simulink subsystem "FTC2019b"  (R2019b)
settings: Solver=VariableStepAuto  StartTime=0.0  StopTime=10.0  RelTol=1e-3
values from neighbouring files (symbols this model uses):
  g = (9.8)    (= 9.8)    [H250_LOEKnown_400HzParam.m]    (also in H250_LOEUnknown_400HzParam.m; H333_LOEKnown_400HzParam.m)
  J = (diag([0.0056 0.0056 0.0104]))    [H250_LOEKnown_400HzParam.m]    (also in H250_LOEUnknown_400HzParam.m; H333_LOEKnown_400HzParam.m = (diag([0.012 0.0120 0.02])))
  m = (0.752)    (= 0.752)    [H250_LOEKnown_400HzParam.m]    (also in H250_LOEUnknown_400HzParam.m; H333_LOEKnown_400HzParam.m = 1.13)
  M = ([ 1          1          1         1 ... (first row only)    [H250_LOEKnown_400HzParam.m]    (also in H250_LOEUnknown_400HzParam.m; H333_LOEKnown_400HzParam.m)
  MY_ATT_P = Pixhawk_CSC.Parameter( {single(8), 'MY_ATT_P'}  )    [H250_LOEKnown_400HzParam.m]    (also in H250_LOEUnknown_400HzParam.m = Pixhawk_CSC.Parameter( {single(3), 'MY_ATT_P'}  ); H333_LOEKnown_400HzParam.m)
  MY_ATT_P_YAW = Pixhawk_CSC.Parameter( {single(0), 'MY_ATT_P_YAW'}  )    [H250_LOEKnown_400HzParam.m]    (also in H250_LOEUnknown_400HzParam.m = Pixhawk_CSC.Parameter( {single(0.0), 'MY_ATT_P_YAW'}  ); H333_LOEKnown_400HzParam.m)
  MY_POS_P = Pixhawk_CSC.Parameter( {single(0.5), 'MY_POS_P'}  )    [H250_LOEKnown_400HzParam.m]    (also in H250_LOEUnknown_400HzParam.m; H333_LOEKnown_400HzParam.m)
  MY_RATE_P = Pixhawk_CSC.Parameter( {single(12), 'MY_RATE_P'}  )    [H250_LOEKnown_400HzParam.m]    (also in H250_LOEUnknown_400HzParam.m = Pixhawk_CSC.Parameter( {single(14), 'MY_RATE_P'}  ); H333_LOEKnown_400HzParam.m)
  MY_RATE_P_YAW = Pixhawk_CSC.Parameter( {single(0.3), 'MY_RATE_P_YAW'}  )    [H250_LOEKnown_400HzParam.m]    (also in H250_LOEUnknown_400HzParam.m = Pixhawk_CSC.Parameter( {single(0.0), 'MY_RATE_P_YAW'}  ); H333_LOEKnown_400HzParam.m)
  MY_SAT_AD = Pixhawk_CSC.Parameter({single(0.13), 'MY_SAT_AD'} )    [H250_LOEKnown_400HzParam.m]    (also in H250_LOEUnknown_400HzParam.m; H333_LOEKnown_400HzParam.m)
  MY_TAU_P_A = Pixhawk_CSC.Parameter( {single(0), 'MY_TAU_P_A'}  )    [H250_LOEKnown_400HzParam.m]    (also in H250_LOEUnknown_400HzParam.m = Pixhawk_CSC.Parameter( {single(0.0), 'MY_TAU_P_A'}  ); H333_LOEKnown_400HzParam.m)
  MY_TAU_P_A_YAW = Pixhawk_CSC.Parameter( {single(0), 'MY_TAU_P_A_YAW'}  )    [H250_LOEKnown_400HzParam.m]    (also in H250_LOEUnknown_400HzParam.m; H333_LOEKnown_400HzParam.m)
  MY_TAU_P_P = Pixhawk_CSC.Parameter( {single(1.5), 'MY_TAU_P_P'}  )    [H250_LOEKnown_400HzParam.m]    (also in H250_LOEUnknown_400HzParam.m = Pixhawk_CSC.Parameter( {single(1.3), 'MY_TAU_P_P'}  ); H333_LOEKnown_400HzParam.m)
  MY_TAU_P_P_YAW = Pixhawk_CSC.Parameter( {single(0.1), 'MY_TAU_P_P_YAW'}  )    [H250_LOEKnown_400HzParam.m]    (also in H250_LOEUnknown_400HzParam.m; H333_LOEKnown_400HzParam.m)
  MY_VEL_P = Pixhawk_CSC.Parameter( {single(0.8), 'MY_VEL_P'}  )    [H250_LOEKnown_400HzParam.m]    (also in H250_LOEUnknown_400HzParam.m; H333_LOEKnown_400HzParam.m)
  T00 = single([m*g/4 m*g/4 m*g/4 m*g/4]')    [H250_LOEKnown_400HzParam.m]    (also in H250_LOEUnknown_400HzParam.m; H333_LOEKnown_400HzParam.m)
  Tf = 0.06    [H250_LOEKnown_400HzParam.m]    (also in H250_LOEUnknown_400HzParam.m; H333_LOEKnown_400HzParam.m)
  Tmotorbar = (0.035)    (= 0.035)    [H250_LOEKnown_400HzParam.m]    (also in H250_LOEUnknown_400HzParam.m = 0.032; H333_LOEKnown_400HzParam.m)
  Ts = 1/400    (= 0.0025)    [H250_LOEKnown_400HzParam.m]    (also in H250_LOEUnknown_400HzParam.m; H333_LOEKnown_400HzParam.m)
libraries: discretizing x8, simulink x1, sharedtransform x1
settings Model: Creator=kcx06  LastModifiedBy=kcx06

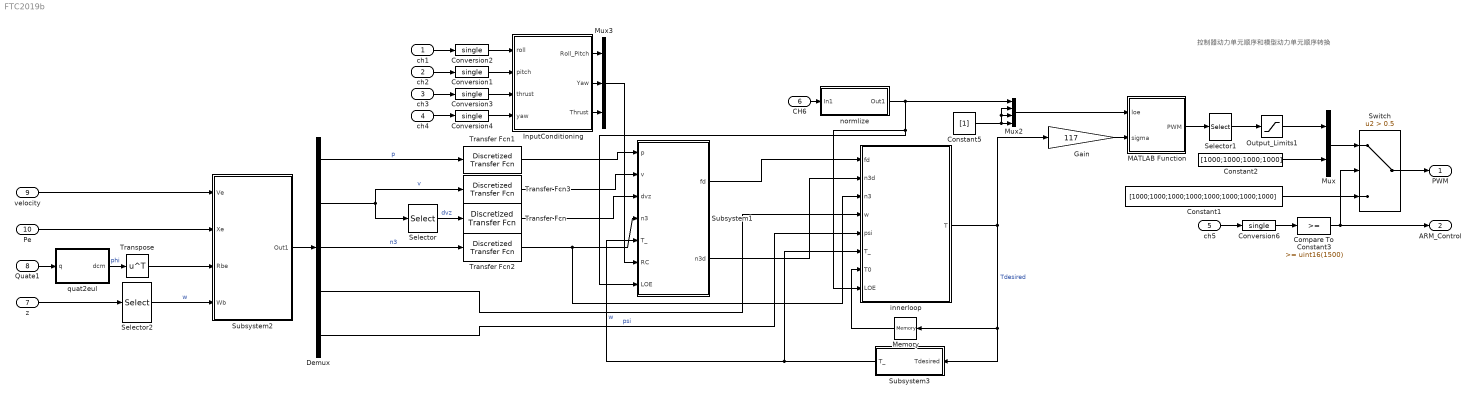
== system FTC2019b ==
  note: 控制器动力单元顺序和模型动力单元顺序转换
  ch1 : Inport  OutDataTypeStr=uint16  PortDimensions=1
  ch2 : Inport  Port=2  OutDataTypeStr=uint16  PortDimensions=1
  ch3 : Inport  Port=3  OutDataTypeStr=uint16  PortDimensions=1
  ch4 : Inport  Port=4  OutDataTypeStr=uint16  PortDimensions=1
  ch5 : Inport  Port=5  OutDataTypeStr=uint16  PortDimensions=1  Interpolate=off
  CH6 : Inport  Port=6
  z : Inport  Port=7
  Quate1 : Inport  Port=8
  velocity : Inport  Port=9
  Pe : Inport  Port=10
  Compare To Constant3 : simulink/Logic and Bit Operations/Compare To Constant  relop=>=  const=uint16(1500)  OutDataTypeStr=boolean
  Constant1 : Constant  Value=[1000;1000;1000;1000;1000;1000;1000;1000]  OutDataTypeStr=single
  Constant2 : Constant  Value=[1000;1000;1000;1000]  OutDataTypeStr=single
  Constant5 : Constant  Value=[1]  OutDataTypeStr=single
  Conversion{1..4,6} (5 alike) : DataTypeConversion  OutDataTypeStr=single
  Demux : Demux  Outputs=[3 3 3 3 1]
  Gain : Gain  Gain=117
  InputConditioning : Subsystem
  MATLAB Function : MATLAB Function  TreatAsAtomicUnit=on
  Memory : Memory  InitialCondition=T00
  Mux : Mux  Inputs=2
  Mux2 : Mux
  Mux3 : Mux  Inputs=3
  Output_Limits1 : Saturate  UpperLimit=2000  LowerLimit=900
  Selector : Selector  IndexMode=Zero-based  InputPortWidth=3  IndexOptions=Index vector (dialog)  Indices=[2]  OutputSizes=1
  Selector1 : Selector  IndexMode=Zero-based  InputPortWidth=4  IndexOptions=Index vector (dialog)  Indices=[0 2 3 1]  OutputSizes=1
  Selector2 : Selector  IndexMode=Zero-based  InputPortWidth=6  IndexOptions=Index vector (dialog)  Indices=[0 1 2]  OutputSizes=1
  Subsystem1 : Subsystem
  Subsystem2 : Subsystem
  Subsystem3 : Subsystem
  Switch : Switch  Criteria=u2 > Threshold  Threshold=0.5
  Transfer Fcn : discretizing/Discretized Transfer Fcn  Numerator=[1 0]  Denominator=[Tf 1]  AbsTol=auto  SampleTime=Ts  method=zoh  Wc=1
      settings: SourceProductBaseCode=SL
  Transfer Fcn1 : discretizing/Discretized Transfer Fcn  Numerator=[1 ]  Denominator=[Tf 1]  AbsTol=auto  SampleTime=Ts  method=zoh  Wc=1
      link override Discrete Transfer Fcn: InitialStates=[0;0;0]
      settings: SourceProductBaseCode=SL
  Transfer Fcn2 : discretizing/Discretized Transfer Fcn  Numerator=[1 ]  Denominator=[Tf 1]  AbsTol=auto  SampleTime=Ts  method=zoh  Wc=1
      link override Discrete Transfer Fcn: InitialStates=[0;0;1]
      settings: SourceProductBaseCode=SL
  Transfer Fcn3 : discretizing/Discretized Transfer Fcn  Numerator=[1 ]  Denominator=[Tf 1]  AbsTol=auto  SampleTime=Ts  method=zoh  Wc=1
      link override Discrete Transfer Fcn: InitialStates=[0;0;0]
      settings: SourceProductBaseCode=SL
  Transpose : Math  Operator=transpose  SaturateOnIntegerOverflow=on
  innerloop : Subsystem
  normlize : Subsystem
  quat2eul : MATLAB Function  TreatAsAtomicUnit=on
  PWM : Outport  PortDimensions=8  VectorParamsAs1DForOutWhenUnconnected=off
  ARM_Control : Outport  Port=2  PortDimensions=1  VectorParamsAs1DForOutWhenUnconnected=off
  wires:
  Compare To Constant3/1 -> ARM_Control/1, Switch/2
  Conversion4/1 -> InputConditioning/4(yaw)
  Output_Limits1/1 -> Mux/1
  ch4/1 -> Conversion4/1
  ch2/1 -> Conversion1/1
  ch5/1 -> Conversion6/1
  Conversion1/1 -> InputConditioning/2(pitch)
  Conversion6/1 -> Compare To Constant3/1
  Conversion2/1 -> InputConditioning/1(roll)
  ch1/1 -> Conversion2/1
  ch3/1 -> Conversion3/1
  Constant2/1 -> Mux/2
  Mux/1 -> Switch/1
  Constant1/1 -> Switch/3
  innerloop/1(T) -> Gain/1, Memory/1, Subsystem3/1(Tdesired)  "Tdesired"
  Demux/5 -> innerloop/5(psi)  "psi"
  Memory/1 -> innerloop/7(T0)
  Selector/1 -> Transfer Fcn/1  "dvz"
  Demux/4 -> innerloop/4(w)  "w"
  Demux/2 -> Transfer Fcn3/1, Selector/1  "v"
  Selector1/1 -> Output_Limits1/1
  Gain/1 -> MATLAB Function/2(sigma)
  MATLAB Function/1(PWM) -> Selector1/1
  Subsystem2/1(Out1) -> Demux/1
  Selector2/1 -> Subsystem2/4(Wb)  "w"
  velocity/1 -> Subsystem2/1(Ve)
  Pe/1 -> Subsystem2/2(Xe)
  Quate1/1 -> quat2eul/1(q)
  Conversion3/1 -> InputConditioning/3(thrust)
  quat2eul/1(dcm) -> Transpose/1  "phi"
  Subsystem1/1(fd) -> innerloop/1(fd)
  Demux/1 -> Transfer Fcn1/1  "p"
  Subsystem1/2(n3d) -> innerloop/2(n3d)
  Subsystem3/1(T_) -> innerloop/6(T_), Subsystem1/5(T_)
  CH6/1 -> normlize/1(In1)
  normlize/1(Out1) -> innerloop/8(LOE), Subsystem1/7(LOE), Mux2/1
  Mux2/1 -> MATLAB Function/1(loe)
  Transfer Fcn/1 -> Subsystem1/3(dvz)
  Constant5/1 -> Mux2/4, Mux2/3, Mux2/2
  Transpose/1 -> Subsystem2/3(Rbe)
  Demux/3 -> Transfer Fcn2/1  "n3"
  InputConditioning/1(Roll_Pitch) -> Mux3/1
  InputConditioning/2(Yaw) -> Mux3/2
  InputConditioning/3(Thrust) -> Mux3/3
  z/1 -> Selector2/1
  Mux3/1 -> Subsystem1/6(RC)
  Switch/1 -> PWM/1
  Transfer Fcn3/1 -> Subsystem1/2(v)
  Transfer Fcn1/1 -> Subsystem1/1(p)
  Transfer Fcn2/1 -> Subsystem1/4(n3), innerloop/3(n3)

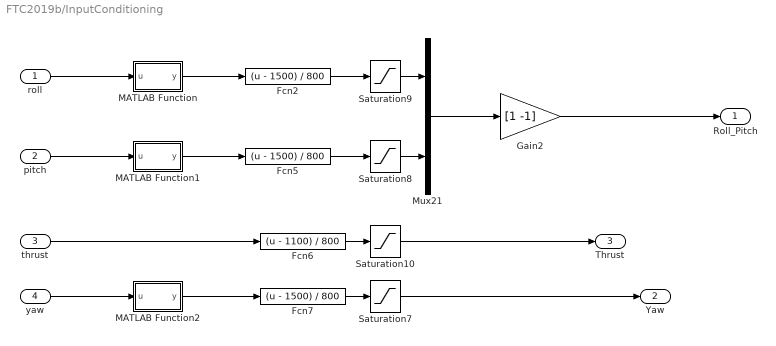
== system FTC2019b/InputConditioning ==
  roll : Inport
  pitch : Inport  Port=2
  thrust : Inport  Port=3
  yaw : Inport  Port=4
  Fcn2 : Fcn  Expr=(u - 1500) / 800
  Fcn5 : Fcn  Expr=(u - 1500) / 800
  Fcn6 : Fcn  Expr=(u - 1100) / 800
  Fcn7 : Fcn  Expr=(u - 1500) / 800
  Gain2 : Gain  Gain=[1 -1]  OutDataTypeStr=Inherit: Inherit via back propagation
  MATLAB Function : MATLAB Function  TreatAsAtomicUnit=on
  MATLAB Function1 : MATLAB Function  TreatAsAtomicUnit=on
  MATLAB Function2 : MATLAB Function  TreatAsAtomicUnit=on
  Mux21 : Mux  Inputs=2
  Saturation10 : Saturate  UpperLimit=1  LowerLimit=0
  Saturation7 : Saturate  UpperLimit=1  LowerLimit=-1
  Saturation8 : Saturate  UpperLimit=1  LowerLimit=-1
  Saturation9 : Saturate  UpperLimit=1  LowerLimit=-1
  Roll_Pitch : Outport  VectorParamsAs1DForOutWhenUnconnected=off
  Yaw : Outport  Port=2  VectorParamsAs1DForOutWhenUnconnected=off
  Thrust : Outport  Port=3  VectorParamsAs1DForOutWhenUnconnected=off
  wires:
  yaw/1 -> MATLAB Function2/1(u)
  MATLAB Function/1(y) -> Fcn2/1
  MATLAB Function1/1(y) -> Fcn5/1
  roll/1 -> MATLAB Function/1(u)
  thrust/1 -> Fcn6/1
  MATLAB Function2/1(y) -> Fcn7/1
  pitch/1 -> MATLAB Function1/1(u)
  Fcn7/1 -> Saturation7/1
  Saturation9/1 -> Mux21/1
  Fcn5/1 -> Saturation8/1
  Fcn2/1 -> Saturation9/1
  Fcn6/1 -> Saturation10/1
  Saturation8/1 -> Mux21/2
  Mux21/1 -> Gain2/1
  Gain2/1 -> Roll_Pitch/1
  Saturation7/1 -> Yaw/1
  Saturation10/1 -> Thrust/1

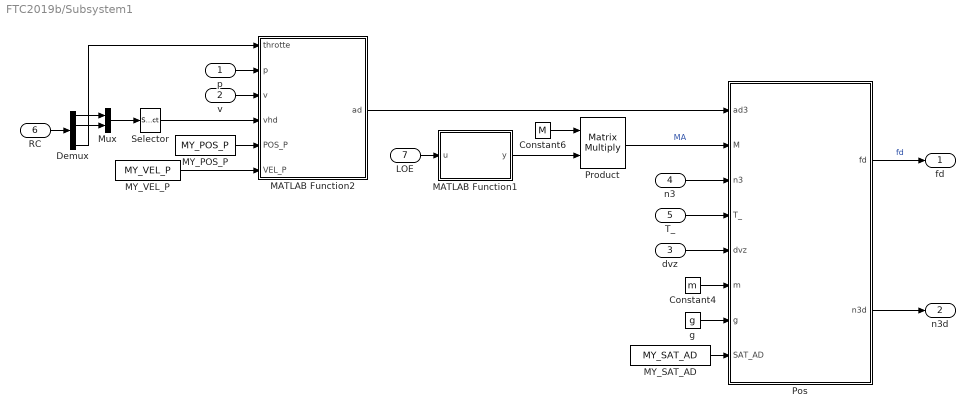
== system FTC2019b/Subsystem1 ==
  p : Inport
  v : Inport  Port=2
  dvz : Inport  Port=3
  n3 : Inport  Port=4
  T_ : Inport  Port=5
  RC : Inport  Port=6
  LOE : Inport  Port=7
  Constant4 : Constant  Value=m  OutDataTypeStr=single
  Constant6 : Constant  Value=M  OutDataTypeStr=single
  Demux : Demux
  MATLAB Function1 : MATLAB Function  TreatAsAtomicUnit=on
  MATLAB Function2 : MATLAB Function  TreatAsAtomicUnit=on
  MY_POS_P : Constant  Value=MY_POS_P
  MY_SAT_AD : Constant  Value=MY_SAT_AD
      settings: AttributesFormatString=|
      | 0.13
      | Default
  MY_VEL_P : Constant  Value=MY_VEL_P
  Mux : Mux  Inputs=2
  Pos : MATLAB Function  TreatAsAtomicUnit=on
  Product : Product  Multiplication=Matrix(*)
  Selector : Selector  IndexMode=Zero-based  InputPortWidth=2  IndexOptions=Index vector (dialog)  Indices=[1 0]  OutputSizes=1
  g : Constant  Value=g  OutDataTypeStr=single
  fd : Outport
  n3d : Outport  Port=2
  wires:
  MY_SAT_AD/1 -> Pos/8(SAT_AD)
  MY_POS_P/1 -> MATLAB Function2/5(POS_P)
  MY_VEL_P/1 -> MATLAB Function2/6(VEL_P)
  Selector/1 -> MATLAB Function2/4(vhd)
  Mux/1 -> Selector/1
  Demux/2 -> Mux/2
  Demux/1 -> Mux/1
  v/1 -> MATLAB Function2/3(v)
  MATLAB Function2/1(ad) -> Pos/1(ad3)
  Demux/4 -> MATLAB Function2/1(throtte)
  RC/1 -> Demux/1
  Product/1 -> Pos/2(M)  "MA"
  Constant6/1 -> Product/1
  LOE/1 -> MATLAB Function1/1(u)
  MATLAB Function1/1(y) -> Product/2
  n3/1 -> Pos/3(n3)
  p/1 -> MATLAB Function2/2(p)
  g/1 -> Pos/7(g)
  Constant4/1 -> Pos/6(m)
  T_/1 -> Pos/4(T_)
  Pos/2(n3d) -> n3d/1
  Pos/1(fd) -> fd/1  "fd"
  dvz/1 -> Pos/5(dvz)

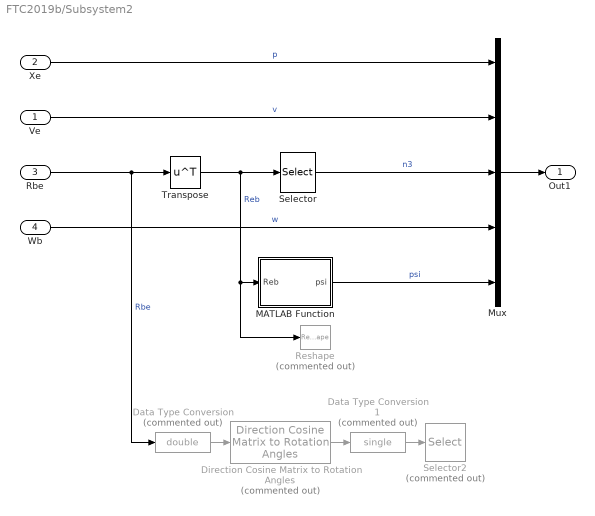
== system FTC2019b/Subsystem2 ==
  Ve : Inport
  Xe : Inport  Port=2
  Rbe : Inport  Port=3
  Wb : Inport  Port=4
  Data Type Conversion : DataTypeConversion  Commented=on  OutDataTypeStr=double
  Data Type Conversion1 : DataTypeConversion  Commented=on  OutDataTypeStr=single
  Direction Cosine Matrix to Rotation Angles : sharedtransform/Direction Cosine Matrix to Rotation Angles  Commented=on  rotationOrder=ZYX  aMode=aMode  action=None  tolerance=eps(2)
      settings: SourceProductBaseCode=AE,PW,MT,UV,VE,VP
  MATLAB Function : MATLAB Function  TreatAsAtomicUnit=on
  Mux : Mux  Inputs=[3 3 3 3 1]
  Reshape : Reshape  Commented=on
  Selector : Selector  NumberOfDimensions=2  IndexMode=Zero-based  InputPortWidth=3  IndexOptions=Select all,Index vector (dialog)  Indices=[1 3],2  OutputSizes=1,1
  Selector2 : Selector  Commented=on  InputPortWidth=3  IndexOptions=Index vector (dialog)  Indices=[3 2 1]  OutputSizes=1
  Transpose : Math  Operator=transpose  SaturateOnIntegerOverflow=on
  Out1 : Outport
  wires:
  Data Type Conversion1/1 -> Selector2/1
  Data Type Conversion/1 -> Direction Cosine Matrix to Rotation Angles/1
  Direction Cosine Matrix to Rotation Angles/1 -> Data Type Conversion1/1
  MATLAB Function/1(psi) -> Mux/5  "psi"
  Wb/1 -> Mux/4  "w"
  Mux/1 -> Out1/1
  Selector/1 -> Mux/3  "n3"
  Transpose/1 -> Selector/1, MATLAB Function/1(Reb), Reshape/1  "Reb"
  Rbe/1 -> Transpose/1, Data Type Conversion/1  "Rbe"
  Ve/1 -> Mux/2  "v"
  Xe/1 -> Mux/1  "p"

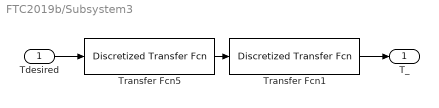
== system FTC2019b/Subsystem3 ==
  Tdesired : Inport
  Transfer Fcn1 : discretizing/Discretized Transfer Fcn  Numerator=[1]  Denominator=[Tmotorbar 1]  AbsTol=auto  SampleTime=Ts  method=zoh  Wc=1
      settings: SourceProductBaseCode=SL
  Transfer Fcn5 : discretizing/Discretized Transfer Fcn  Numerator=[1]  Denominator=[Tf 1]  AbsTol=auto  SampleTime=Ts  method=zoh  Wc=1
      settings: SourceProductBaseCode=SL
  T_ : Outport
  wires:
  Tdesired/1 -> Transfer Fcn5/1
  Transfer Fcn1/1 -> T_/1
  Transfer Fcn5/1 -> Transfer Fcn1/1

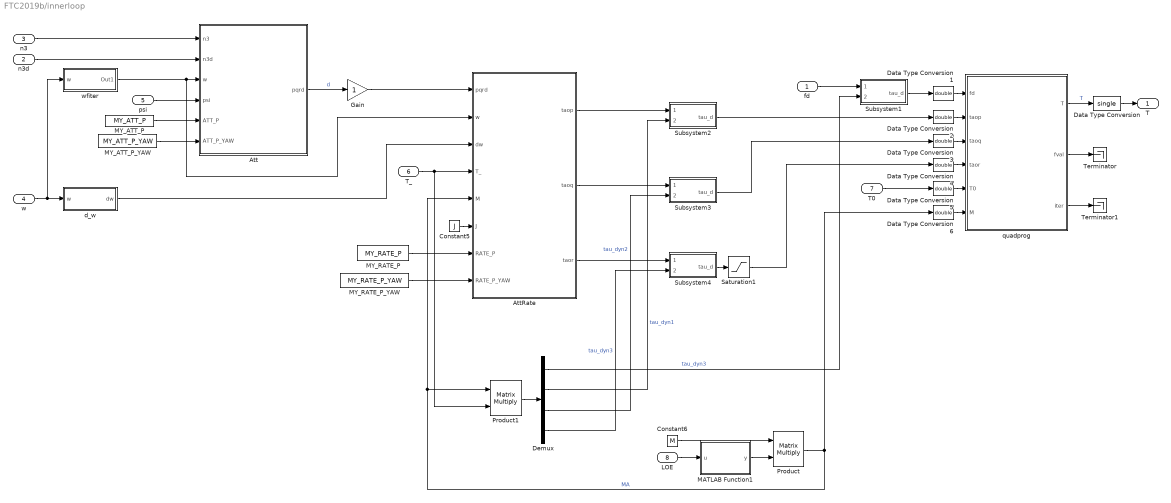
== system FTC2019b/innerloop ==
  fd : Inport
  n3d : Inport  Port=2
  n3 : Inport  Port=3
  w : Inport  Port=4
  psi : Inport  Port=5
  T_ : Inport  Port=6
  T0 : Inport  Port=7
  LOE : Inport  Port=8
  Att : MATLAB Function  TreatAsAtomicUnit=on
  AttRate : MATLAB Function  TreatAsAtomicUnit=on
  Constant5 : Constant  Value=J  OutDataTypeStr=single
  Constant6 : Constant  Value=M  OutDataTypeStr=single
  Data Type Conversion : DataTypeConversion  OutDataTypeStr=single
  Data Type Conversion{1..6} (6 alike) : DataTypeConversion  OutDataTypeStr=double
  Demux : Demux
  Gain : Gain  OutDataTypeStr=single
  MATLAB Function1 : MATLAB Function  TreatAsAtomicUnit=on
  MY_ATT_P : Constant  Value=MY_ATT_P
  MY_ATT_P_YAW : Constant  Value=MY_ATT_P_YAW
  MY_RATE_P : Constant  Value=MY_RATE_P
  MY_RATE_P_YAW : Constant  Value=MY_RATE_P_YAW
  Product : Product  Multiplication=Matrix(*)
  Product1 : Product  Multiplication=Matrix(*)
  Saturation1 : Saturate  UpperLimit=0.075  LowerLimit=-0.075
  Subsystem1 : Subsystem
  Subsystem2 : Subsystem
  Subsystem3 : Subsystem
  Subsystem4 : Subsystem
  Terminator : Terminator
  Terminator1 : Terminator
  d_w : Subsystem
  quadprog : MATLAB Function  TreatAsAtomicUnit=on
  wfiter : Subsystem
  T : Outport  PortDimensions=4
  wires:
  quadprog/3(iter) -> Terminator1/1
  Subsystem4/1(tau_d) -> Saturation1/1
  Subsystem3/1(tau_d) -> Data Type Conversion3/1
  Subsystem2/1(tau_d) -> Data Type Conversion2/1
  n3d/1 -> Att/2(n3d)
  MY_ATT_P_YAW/1 -> Att/6(ATT_P_YAW)
  MY_ATT_P/1 -> Att/5(ATT_P)
  MY_RATE_P_YAW/1 -> AttRate/8(RATE_P_YAW)
  MY_RATE_P/1 -> AttRate/7(RATE_P)
  Data Type Conversion/1 -> T/1
  MATLAB Function1/1(y) -> Product/2
  Att/1(pqrd) -> Gain/1  "d"
  Product1/1 -> Demux/1
  n3/1 -> Att/1(n3)
  Product/1 -> AttRate/5(M), Product1/1, Data Type Conversion6/1  "MA"
  LOE/1 -> MATLAB Function1/1(u)
  Saturation1/1 -> Data Type Conversion4/1
  Demux/4 -> Subsystem4/2(tau_dyn)  "tau_dyn3"
  Demux/3 -> Subsystem3/2(tau_dyn)  "tau_dyn2"
  Demux/2 -> Subsystem2/2(tau_dyn)  "tau_dyn1"
  fd/1 -> Subsystem1/1(tau_dynd)
  Demux/1 -> Subsystem1/2(tau_dyn)  "tau_dyn3"
  Gain/1 -> AttRate/1(pqrd)
  Subsystem1/1(tau_d) -> Data Type Conversion1/1
  AttRate/3(taor) -> Subsystem4/1(tau_dynd)
  AttRate/2(taoq) -> Subsystem3/1(tau_dynd)
  AttRate/1(taop) -> Subsystem2/1(tau_dynd)
  Data Type Conversion6/1 -> quadprog/6(M)
  Data Type Conversion5/1 -> quadprog/5(T0)
  Data Type Conversion4/1 -> quadprog/4(taor)
  Data Type Conversion3/1 -> quadprog/3(taoq)
  Data Type Conversion2/1 -> quadprog/2(taop)
  Data Type Conversion1/1 -> quadprog/1(fd)
  quadprog/1(T) -> Data Type Conversion/1  "T"
  wfiter/1(Out1) -> Att/3(w), AttRate/2(w)
  w/1 -> wfiter/1(w), d_w/1(w)
  psi/1 -> Att/4(psi)
  quadprog/2(fval) -> Terminator/1
  Constant6/1 -> Product/1
  Constant5/1 -> AttRate/6(J)
  T_/1 -> AttRate/4(T_), Product1/2
  T0/1 -> Data Type Conversion5/1
  d_w/1(dw) -> AttRate/3(dw)

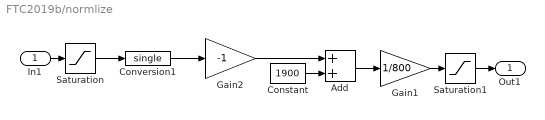
== system FTC2019b/normlize ==
  In1 : Inport
  Add : Sum
  Constant : Constant  Value=1900  OutDataTypeStr=single
  Conversion1 : DataTypeConversion  OutDataTypeStr=single
  Gain1 : Gain  Gain=1/800
  Gain2 : Gain  Gain=-1
  Saturation : Saturate  UpperLimit=1900  LowerLimit=1100
  Saturation1 : Saturate  UpperLimit=1  LowerLimit=0
  Out1 : Outport
  wires:
  Saturation1/1 -> Out1/1
  Conversion1/1 -> Gain2/1
  Constant/1 -> Add/2
  In1/1 -> Saturation/1
  Add/1 -> Gain1/1
  Gain1/1 -> Saturation1/1
  Gain2/1 -> Add/1
  Saturation/1 -> Conversion1/1

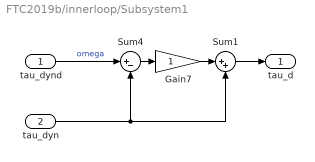
== system FTC2019b/innerloop/Subsystem1 ==
  tau_dynd : Inport
  tau_dyn : Inport  Port=2
  Gain7 : Gain
  Sum1 : Sum  Inputs=|++
  Sum4 : Sum  Inputs=|+-
  tau_d : Outport
  wires:
  tau_dyn/1 -> Sum4/2, Sum1/2
  Sum1/1 -> tau_d/1
  Sum4/1 -> Gain7/1
  Gain7/1 -> Sum1/1
  tau_dynd/1 -> Sum4/1  "omega"

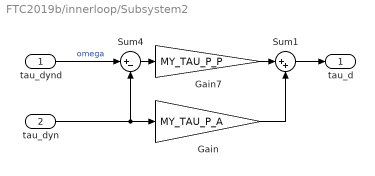
== system FTC2019b/innerloop/Subsystem2 ==
  tau_dynd : Inport
  tau_dyn : Inport  Port=2
  Gain : Gain  Gain=MY_TAU_P_A
  Gain7 : Gain  Gain=MY_TAU_P_P
  Sum1 : Sum  Inputs=|++
  Sum4 : Sum  Inputs=|+-
  tau_d : Outport
  wires:
  Gain/1 -> Sum1/2
  tau_dynd/1 -> Sum4/1  "omega"
  Gain7/1 -> Sum1/1
  Sum4/1 -> Gain7/1
  Sum1/1 -> tau_d/1
  tau_dyn/1 -> Gain/1, Sum4/2

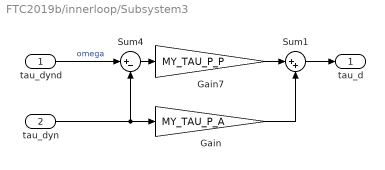
== system FTC2019b/innerloop/Subsystem3 ==
  tau_dynd : Inport
  tau_dyn : Inport  Port=2
  Gain : Gain  Gain=MY_TAU_P_A
  Gain7 : Gain  Gain=MY_TAU_P_P
  Sum1 : Sum  Inputs=|++
  Sum4 : Sum  Inputs=|+-
  tau_d : Outport
  wires:
  tau_dyn/1 -> Sum4/2, Gain/1
  tau_dynd/1 -> Sum4/1  "omega"
  Gain/1 -> Sum1/2
  Sum1/1 -> tau_d/1
  Sum4/1 -> Gain7/1
  Gain7/1 -> Sum1/1

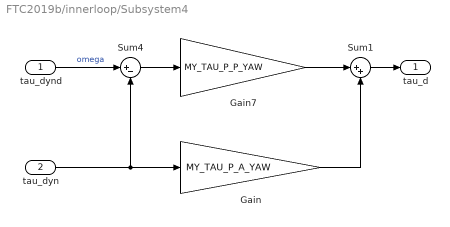
== system FTC2019b/innerloop/Subsystem4 ==
  tau_dynd : Inport
  tau_dyn : Inport  Port=2
  Gain : Gain  Gain=MY_TAU_P_A_YAW
  Gain7 : Gain  Gain=MY_TAU_P_P_YAW
  Sum1 : Sum  Inputs=|++
  Sum4 : Sum  Inputs=|+-
  tau_d : Outport
  wires:
  Gain/1 -> Sum1/2
  tau_dynd/1 -> Sum4/1  "omega"
  Gain7/1 -> Sum1/1
  Sum4/1 -> Gain7/1
  Sum1/1 -> tau_d/1
  tau_dyn/1 -> Gain/1, Sum4/2

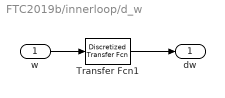
== system FTC2019b/innerloop/d_w ==
  w : Inport
  Transfer Fcn1 : discretizing/Discretized Transfer Fcn  Numerator=[1 0]  Denominator=[Tf 1]  AbsTol=auto  SampleTime=Ts  method=zoh  Wc=1
      settings: SourceProductBaseCode=SL
  dw : Outport
  wires:
  Transfer Fcn1/1 -> dw/1
  w/1 -> Transfer Fcn1/1

== system FTC2019b/innerloop/wfiter ==
  w : Inport
  Transfer Fcn1 : discretizing/Discretized Transfer Fcn  Numerator=[1]  Denominator=[Tf 1]  AbsTol=auto  SampleTime=Ts  method=zoh  Wc=1
      settings: SourceProductBaseCode=SL
  Out1 : Outport
  wires:
  Transfer Fcn1/1 -> Out1/1
  w/1 -> Transfer Fcn1/1

== matlab function FTC2019b/InputConditioning/MATLAB Function ==
  data: u input; y output
function y = fcn(u)

 if(u>1550)
    y=u;
 else
     if(u<1450)
     y=u;
     else
         y=single(1500);
     end
 end

== matlab function FTC2019b/InputConditioning/MATLAB Function1 ==
  data: u input; y output
function y = fcn(u)

 if(u>1550)
    y=u;
 else
     if(u<1450)
     y=u;
     else
         y=single(1500);
     end
 end

== matlab function FTC2019b/InputConditioning/MATLAB Function2 ==
  data: u input; y output
function y = fcn(u)

 if(u>1550)
    y=u;
 else
     if(u<1450)
     y=u;
     else
         y=single(1500);
     end
 end

== matlab function FTC2019b/MATLAB Function ==
  data: loe input; PWM output; sigma input
function PWM = fcn(loe, sigma)
y = loe.*sigma + 1000;
if loe(1) <= 0.1
    y(1) = y(1)-200;
end
PWM = y;

== matlab function FTC2019b/Subsystem1/MATLAB Function1 ==
  data: u input; y output
function y = fcn(u)
y=diag([u,1,1,1]);

== matlab function FTC2019b/Subsystem1/MATLAB Function2 ==
  data: throtte input; ad output; p input; v input; vhd input; POS_P input; VEL_P input
function ad = fcn(throtte, p, v, vhd, POS_P, VEL_P)
persistent pd
if isempty(pd)
    pd = single(p);
end
%% 高度通道
if throtte>=0.4&& throtte <=0.6
        vd3 = mysatsingle(POS_P * (pd(3) - p(3)), 0.5);
        ad3 = VEL_P * (vd3 - v(3));
else
    if throtte>0.6
        vd3 = -1;
        ad3 = VEL_P * (vd3 - v(3));
        pd(3) = p(3);
    else
        vd3 = 1;
        ad3 = VEL_P * (vd3 - v(3));
        pd(3) = p(3);
    end
end
%% 水平通道
if norm(vhd) <= 0.05
        vd12 = mysatsingle(POS_P * (pd(1:2) - p(1:2)), 0.5);
        ad12 = VEL_P * (vd12 - v(1:2));
else
        vd12 = mysatsingle(5*vhd, 0.7);
        ad12 = VEL_P * (vd12 - v(1:2));
        pd(1:2) = p(1:2);
end
ad = [ad12;ad3];

== matlab function FTC2019b/Subsystem1/Pos ==
  data: ad3 input single size=[3,1]; M input; n3 input; T_ input; dvz input; m input single size=1; fd output single size=1; g input single size=1; n3d output single size=3; SAT_AD input
function [fd, n3d]  = fcn(ad3, M, n3,  T_, dvz, m, g, SAT_AD)
ad = mysatsingle(ad3, single(SAT_AD)*g);
n3d = ([single(0); single(0); g]-ad)/norm([single(0); single(0); g]-ad);
if n3d(3)==single(0)
    fd = single(0);
else
    fd = (-ad(3) + dvz)*m/n3(3)+M(1,:)*T_;
end

== matlab function FTC2019b/Subsystem2/MATLAB Function ==
  data: Reb input; psi output
function psi = fcn(Reb)
psi = atan2(Reb(2,1), Reb(1,1));

== matlab function FTC2019b/innerloop/Att ==
  data: n3 input; n3d input; w input; psi input; pqrd output; ATT_P input; ATT_P_YAW input
function pqrd  = fcn(n3, n3d, w, psi, ATT_P, ATT_P_YAW)
%% 角度控制1
% h1 = n3(1);
% h2 = n3(2);
% h3 = n3(3);
% h1d = n3d(1);
% h2d = n3d(2);
% h3d = n3d(3);
% we = Reb*w;
% k1 = single(5);
% epqd = [0 -1/h3; 1/h3 0]*[k1*(h1d-h1)+h2*we(3);k1*(h2d-h2)-h1*we(3)];
% 
% psid = single(0);
% rd = k1*0.3*(psid - psi);
% 
% Rbe = Reb';
% erd = (rd - Rbe(3,1)*epqd(1) - Rbe(3,2)*epqd(2))/Rbe(3,3);
% 
% pqd = Rbe((1:2),:)*[epqd; erd];%计算出机体系下的pqd
% pqd = mysat(pqd,2);
% pqrd = [pqd;rd];
%% 角度控制2
e1  = n3(1) - n3d(1);
e2  = n3(2) - n3d(2); 
beta = atan2(e2,e1);

k1 = ATT_P;
pqd = [ -k1*sqrt(e1^2+e2^2)*sin(psi-beta);
             -k1*sqrt(e1^2+e2^2)*cos(psi-beta);];
pqd = mysatsingle(pqd,2);
psid = 0;
   rd = -k1*ATT_P_YAW*(psi-psid);
% rd = 0;
pqrd = [pqd;rd];

== matlab function FTC2019b/innerloop/AttRate ==
  data: pqrd input; w input; dw input; T_ input; M input; J input; taop output; taoq output; taor output; RATE_P input; RATE_P_YAW input
function [taop, taoq, taor] = fcn(pqrd, w, dw, T_, M, J, RATE_P, RATE_P_YAW)
pqd = pqrd(1:2);
rd    = pqrd(3);
%% 角速率控制器计算
k2 = RATE_P;
taop =           J(1,1)*(k2*(pqd(1)-w(1))) + M(2,:)*T_ -J(1,1)*dw(1);
taoq =           J(2,2)*(k2*(pqd(2)-w(2))) + M(3,:)*T_ -J(2,2)*dw(2);
taor  = mysatsingle(J(3,3)*k2*RATE_P_YAW*(rd-w(3)) + M(4,:)*T_ -J(3,3)*dw(3),20.0);

== matlab function FTC2019b/innerloop/MATLAB Function1 ==
  data: u input; y output
function y = fcn(u)
y=diag([u,1,1,1]);

== matlab function FTC2019b/innerloop/quadprog ==
  data: fd input double; taop input double; taoq input double; taor input double; T output double; T0 input double; M input double; fval output double; iter output
function [T,fval, iter] = fcn(fd, taop, taoq, taor, T0, M)
%% 求解
vd = [fd; taop; taoq; taor];
W=diag([1 20 20 0.9]);
H = M'*W*M;
f = -(vd'*W*M)';
% Td = B*vd;
lb  = [0 0 0 0]';
ub  = [8.5 8.5 8.5 8.5]';
% if (max(B*vd)>3)||(min(B*vd)<0)
    options = optimoptions(@quadprog,'Algorithm','active-set','MaxIterations',5);

    [T,fval,~,output] = quadprog(H, f, [], [], [], [], lb, ub, T0, options);
     iter = output.iterations;
% else
%     T = B*vd;
%     fval = 0;
% end

== matlab function FTC2019b/quat2eul ==
  data: q input single; dcm output single
function dcm  = quat2eul(q)
% Conversion from Quaternion to Euler angles based on the PX4 Firmware
% v1.6.5 release.
% 
% Quaternion -> DCM -> Euler Angles
% INPUT:
%   q: Quaternion vector of the format: (a + bi + cj + dk)
% OUTPUT:
%   [phi,theta,psi]: Euler angles in radians.
% 
 if norm(q)~=0
    a = q(1);
    b = q(2);
    c = q(3);
    d = q(4);

    aSq = a*a;
    bSq = b*b;
    cSq = c*c;
    dSq = d*d;

    d_pi2 = pi/2;

    % quaternion_to_dcm
    dcm00 = aSq + bSq - cSq - dSq;
    dcm01 = 2*(b*c - a*d);
    dcm02 = 2*(a*c + b*d);
    dcm10 = 2*(b*c + a*d);
    dcm11 = aSq - bSq + cSq - dSq;
    dcm12 = 2*(c*d - a*b);
    dcm20 = 2*(b*d - a*c);
    dcm21 = 2*(a*b + c*d);
    dcm22 = aSq - bSq - cSq + dSq;
    dcm=[dcm00 dcm01 dcm02;
              dcm10 dcm11 dcm12;
              dcm20 dcm21  dcm22];
 else
     dcm = single(eye(3,3));
 end
    % dcm_to_euler
